simulink model "w2_warplab_trigger_proc"  (Simulink 7.7)
settings: Solver=ode45  StartTime=0.0  StopTime=1000  RelTol=1e-3
InitFcn:
  | w2_warplab_trigger_proc_init
StartFcn:
  | w2_warplab_trigger_proc_init
undefined symbols (not defined in the file or in its folder): gcbh, xlBlockLoadCallback, xlGetNormalizedPeriod
libraries: xbsIndex_r4 x819, simulink x1
(part 1 of 6)
settings Model: Creator=murphpo  LastModifiedBy=mango
settings DebuggingCC: FcnCallInpInsideContextMsg=Enable All

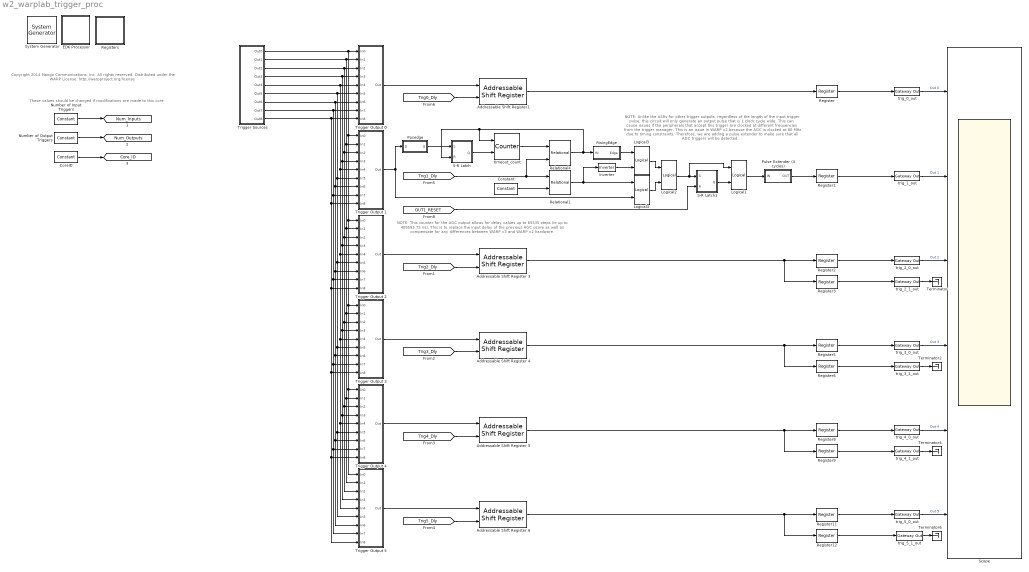
== system w2_warplab_trigger_proc ==
  note: These values should be changed if modifications are made to this core
  note: Copyright 2014 Mango Communications, Inc. All rights reserved.
      |
      | Distributed under the WARP License:
      | http://warpproject.org/license
  note: NOTE:  This counter for the AGC output allows for delay values up to 65535 steps (ie up to 409593.75 ns).
      | This is to replace the input delay of the previous AGC pcore as well as compensate for any differences
      | between WARP v3 and WARP v2 hardware.
  note: NOTE:  Unlike the ASRs for other trigger outputs, regardless of the length of the input trigger pulse, this
      | circuit will only generate an output pulse that is 1 clock cycle wide. This can cause issues if the peripherals
      | that accept this trigger are clocked at different frequencies from the trigger manager.
      |
      | This is an issue in WARP v2 because the AGC is clocked at 80 MHz due to timing constraints.  Therefore,
      | we are adding a pulse extender to make sure that all AGC triggers will be detected.
  " System Generator" : xbsIndex_r4/ System Generator  Tag=genX  SystemSampleTime=-1  xilinxfamily=virtex4  part=xc4vfx100  speed=-11  package=ff1517  synthesis_tool=XST  clock_wrapper=Clock Enables  directory=./trigger_proc  proj_type=Project Navigator  Synth_file=XST Defaults  Impl_file=ISE Defaults  testbench=off  simulink_period=1  sysclk_period=10  dcm_input_clock_period=10  incr_netlist=off  trim_vbits=Everywhere in SubSystem  dbl_ovrd=According to Block Masks  core_generation=According to Block Masks  run_coregen=off  deprecated_control=off  eval_field=0  block_type=sysgen
  Addressable Shift Register {3..6} (4 alike) : xbsIndex_r4/Addressable Shift Register  infer_latency=off  depth=32  initVector=[0]  en=off  dbl_ovrd=off  use_behavioral_HDL=off  Optimization=Resource  block_type=addrsr
      settings: infoedit="Delay of configurable length.  Any element in the delay line can be addressed and driven onto the output port.<br><br>Hardware notes: This block is implemented using SRL16s. If Virtex-4 or Spartan-3 device is used, multiple SRLC16s are cascaded together."
  Addressable Shift Register1 : xbsIndex_r4/Addressable Shift Register  infer_latency=off  depth=32  initVector=[0]  en=off  dbl_ovrd=off  use_behavioral_HDL=off  Optimization=Resource  block_type=addrsr
      settings: infoedit="Delay of configurable length.  Any element in the delay line can be addressed and driven onto the output port.<br><br>Hardware notes: This block is implemented using SRL16s. If Virtex-4 or Spartan-3 device is used, multiple SRLC16s are cascaded together."
  Constant : xbsIndex_r4/Constant  const=0  gui_display_data_type=Fixed-point  arith_type=Unsigned  n_bits=16  bin_pt=0  preci_type=Single  exp_width=8  frac_width=24  explicit_period=off  period=1  equ=P=C  opselect=C  inp2=PCIN>>17  opr=+  inp1=P  carry=CIN  dbl_ovrd=off  block_type=constant
  CoreID : xbsIndex_r4/Constant  const=0  gui_display_data_type=Fixed-point  arith_type=Unsigned  n_bits=8  bin_pt=0  preci_type=Single  exp_width=8  frac_width=24  explicit_period=on  period=1  equ=P=C  opselect=C  inp2=PCIN>>17  opr=+  inp1=P  carry=CIN  dbl_ovrd=off  block_type=constant
  EDK Processor : Subsystem  LoadFcn=xlBlockLoadCallback(gcbh);  mask(Xilinx EDK Processor Block){mode=EDK pcore generation, xmp=, MemVisToProc=<qt bgcolor="#FFFFFF"><div><img src="C:/Xilinx/14.4/ISE_DS/ISE/sysgen/data/images/registerplus.gif"> &lt;&lt;RSSI_PKT_DET_CONFIG&gt;&gt;<br></div><div><img src="C:/Xilinx/14.4/ISE_DS/ISE/sysgen/data/images/registerplus.gif"> &lt;&lt;TRIG_IN_CONF_6&gt;&gt;<br></div><div><img src="C:/Xilinx/14.4/ISE_DS/ISE/sysgen/data/images/registerplus.gif"> &lt;&lt;TRIG_IN_CONF_5&gt;&gt;<br></div><div><img src="C:/Xilinx/14.4/ISE_DS/ISE/sysgen/data/images/registerplus.gif"> &lt;&lt;TRIG_IN_CONF_4&gt;&gt;<br></div><div><img src="C:/Xilinx/14.4/ISE_DS/ISE/sysgen/data/images/registerplus.gif"> &lt;&lt;TRIG_IN_CONF_3&gt;&gt;<br></div><div><img src="C:/Xilinx/14.4/ISE_DS/ISE/sysgen/data/images/registerplus.gif"> &lt;&lt;TRIG_IN_CONF_2&gt;&gt;<br></div><div><img src="C:/Xilinx/14.4/ISE_DS/ISE/sysgen/data/images/registerplus.gif"> &lt;&lt;TRIG_IN_CONF_0&gt;&gt;<br></div><div><img src="C:/Xilinx/14.4/ISE_DS/ISE/sysgen/data/images/registerplus.gif"> &lt;&lt;TRIG_IN_CONF_8&gt;&gt;<br></div><div><img src="C:/Xilinx/14.4/ISE_DS/ISE/sysgen/data/images/registerplus.gif"> &lt;&lt;TRIG_IN_CONF_7&gt;&gt;<br></div><div><img src="C:/Xilinx/14.4/ISE_DS/ISE/sysgen/data/images/registerplus.gif"> &lt;&lt;TRIG_OUT_5_CONF_0&gt;&gt;<br></div><div><img src="C:/Xilinx/14.4/ISE_DS/ISE/sysgen/data/images/registerplus.gif"> &lt;&lt;TRIG_OUT_5_CONF_1&gt;&gt;<br></div><div><img src="C:/Xilinx/14.4/ISE_DS/ISE/sysgen/data/images/registerplus.gif"> &lt;&lt;TRIG_OUT_4_CONF_0&gt;&gt;<br></div><div><img src="C:/Xilinx/14.4/ISE_DS/ISE/sysgen/data/images/registerplus.gif"> &lt;&lt;TRIG_OUT_0_CONF_0&gt;&gt;<br></div><div><img src="C:/Xilinx/14.4/ISE_DS/ISE/sysgen/data/images/registerplus.gif"> &lt;&lt;TRIG_OUT_4_CONF_1&gt;&gt;<br></div><div><img src="C:/Xilinx/14.4/ISE_DS/ISE/sysgen/data/images/registerplus.gif"> &lt;&lt;TRIG_OUT_3_CONF_0&gt;&gt;<br></div><div><img src="C:/Xilinx/14.4/ISE_DS/ISE/sysgen/data/images/registerplus.gif"> &lt;&lt;TRIG_OUT_3_CONF_1&gt;&gt;<br></div><div><img src="C:/Xilinx/14.4/ISE_DS/ISE/sysgen/data/images/registerplus.gif"> &lt;&lt;TRIG_OUT_2_CONF_0&gt;&gt;<br></div><div><img src="C:/Xilinx/14.4/ISE_DS/ISE/sysgen/data/images/registerplus.gif"> &lt;&lt;TRIG_OUT_2_CONF_1&gt;&gt;<br></div><div><img src="C:/Xilinx/14.4/ISE_DS/ISE/sysgen/data/images/registerplus.gif"> &lt;&lt;TRIG_OUT_1_CONF_0&gt;&gt;<br></div><div><img src="C:/Xilinx/14.4/ISE_DS/ISE/sysgen/data/images/registerplus.gif"> &lt;&lt;TRIG_OUT_1_CONF_1&gt;&gt;<br></div><div><img src="C:/Xilinx/14.4/ISE_DS/ISE/sysgen/data/images/registerplus.gif"> &lt;&lt;TRIG_OUT_0_CONF_1&gt;&gt;<br></div><div><img src="C:/Xilinx/14.4/ISE_DS/ISE/sysgen/data/images/registerplus.gif"> &lt;&lt;RSSI_PKT_DET_DURATIONS&gt;&gt;<br></div><div><img src="C:/Xilinx/14.4/ISE_DS/ISE/sysgen/data/images/registerplus.gif"> &lt;&lt;RSSI_PKT_DET_THRESHOLDS&gt;&gt;<br></div><div><img src="C:/Xilinx/14.4/ISE_DS/ISE/sysgen/data/images/registerplus.gif"> &lt;&lt;TRIG_IN_CONF_1&gt;&gt;<br></div><div><img src="C:/Xilinx/14.4/ISE_DS/ISE/sysgen/data/images/registerplus.gif"> &lt;&lt;CORE_INFO&gt;&gt;<br></div><div><img src="C:/Xilinx/14.4/ISE_DS/ISE/sysgen/data/images/registerplus.gif"> &lt;&lt;TRIG_OUT&gt;&gt;<br></div></qt>, AvailableMemories=<empty>, portInterfaceTable={'exposed'=>[],'portdir'=>[],'portname'=>[],'shortname'=>[]}, bus_type_sgadvanced=, bus_type=PLB, baseaddr=0x80000000, baseaddr_lock_sgadvanced=, baseaddr_lock=off, dual_clock_sgadvanced=, dual_clock=on, reg_readback_sgadvanced=, reg_readback=on, ucf_file=, inheritDeviceType_sgadvanced=, inheritDeviceType=off, elf_file=, codebug_sgadvanced=, codebug=on, clock_name=plb, internalPortList={}, resetPolarity=0, memxtable={'mladdr'=>[0.00000000000000000,1.00000000000000000,2.00000000000000000,3.00000000000000000,4.00000000000000000,5.00000000000000000,6.00000000000000000,7.00000000000000000,8.00000000000000000,9.00000000000000000,10.00000000000000000,11.00000000000000000,12.00000000000000000,13.00000000000000000,14.00000000000000000,15.00000000000000000,16.00000000000000000,17.00000000000000000,18.00000000000000000,19.00000000000000000,20.00000000000000000,21.00000000000000000,22.00000000000000000,23.00000000000000000,0.00000000000000000,1.00000000000000000],'mlist'=>['w2_warplab_trigger_proc/Registers/From Register9','w2_warplab_trigger_proc/Registers/From Register8','w2_warplab_trigger_proc/Registers/From Register7','w2_warplab_trigger_proc/Registers/From Register6','w2_warplab_trigger_proc/Registers/From Register5','w2_warplab_trigger_proc/Registers/From Register4','w2_warplab_trigger_proc/Registers/From Register3','w2_warplab_trigger_proc/Registers/From Register24','w2_warplab_trigger_proc/Registers/From Register23','w2_warplab_trigger_proc/Registers/From Register22','w2_warplab_trigger_proc/Registers/From Register21','w2_warplab_trigger_proc/Registers/From Register20','w2_warplab_trigger_proc/Registers/From Register2','w2_warplab_trigger_proc/Registers/From Register19','w2_warplab_trigger_proc/Registers/From Register18','w2_warplab_trigger_proc/Registers/From Register17','w2_warplab_trigger_proc/Registers/From Register16','w2_warplab_trigger_proc/Registers/From Register15','w2_warplab_trigger_proc/Registers/From Register14','w2_warplab_trigger_proc/Registers/From Register13','w2_warplab_trigger_proc/Registers/From Register12','w2_warplab_trigger_proc/Registers/From Register11','w2_warplab_trigger_proc/Registers/From Register10','w2_warplab_trigger_proc/Registers/From Register1','w2_warplab_trigger_proc/Registers/To Register1','w2_warplab_trigger_proc/Registers/To Register'],'mlname'=>['\\'RSSI_PKT_DET_CONFIG\\'','\\'TRIG_IN_CONF_6\\'','\\'TRIG_IN_CONF_5\\'','\\'TRIG_IN_CONF_4\\'','\\'TRIG_IN_CONF_3\\'','\\'TRIG_IN_CONF_2\\'','\\'TRIG_IN_CONF_0\\'','\\'TRIG_IN_CONF_8\\'','\\'TRIG_IN_CONF_7\\'','\\'TRIG_OUT_5_CONF_0\\'','\\'TRIG_OUT_5_CONF_1\\'','\\'TRIG_OUT_4_CONF_0\\'','\\'TRIG_OUT_0_CONF_0\\'','\\'TRIG_OUT_4_CONF_1\\'','\\'TRIG_OUT_3_CONF_0\\'','\\'TRIG_OUT_3_CONF_1\\'','\\'TRIG_OUT_2_CONF_0\\'','\\'TRIG_OUT_2_CONF_1\\'','\\'TRIG_OUT_1_CONF_0\\'','\\'TRIG_OUT_1_CONF_1\\'','\\'TRIG_OUT_0_CONF_1\\'','\\'RSSI_PKT_DET_DURATIONS\\'','\\'RSSI_PKT_DET_THRESHOLDS\\'','\\'TRIG_IN_CONF_1\\'','\\'CORE_INFO\\'','\\'TRIG_OUT\\''],'mlstate'=>[0.00000000000000000,0.00000000000000000,0.00000000000000000,0.00000000000000000,0.00000000000000000,0.00000000000000000,0.00000000000000000,0.00000000000000000,0.00000000000000000,0.00000000000000000,0.00000000000000000,0.00000000000000000,0.00000000000000000,0.00000000000000000,0.00000000000000000,0.00000000000000000,0.00000000000000000,0.00000000000000000,0.00000000000000000,0.00000000000000000,0.00000000000000000,0.00000000000000000,0.00000000000000000,0.00000000000000000,0.00000000000000000,0.00000000000000000]}, procinfo={}, memmapdirty=off, blockname=, xpsintstyle=default, has_advanced_control=0, sggui_pos=-1,-1,-1,-1, block_type=edkprocessor, block_version=2.7, sg_icon_stat=62,64,-1,-1,white,blue,0,07734,right,,[ ],[ ], sg_mask_display=|, sg_list_contents={'table'=>{'AvailableMemories'=>'popup(<empty>)'}}, sg_blockgui_xml=}
      mask sg_mask_display=|
      | fprintf('','COMMENT: begin icon graphics');
      | patch([0 62 62 0 0 ],[0 0 64 64 0 ],[0.77 0.82 0.91 ]);
      | plot([0 62 62 0 0 ],[0 0 64 64 0 ]);
      | patch([13.2 24.76 32.76 40.76 48.76 32.76 21.2 13.2 ],[40.88 40.88 48.88 40.88 48.88 48.88 48.88 40.88 ],[1 1 1 ]);
      | patch([21.2 32.76 24.76 13.2 21.2 ],[32.88 32.88 40.88 40.88 32.88 ],[0.931 0.946 0.973 ]);
      | patch([13.2 24.76 32.76 21.2 13.2 ],[24.88 24.88 32.88 32.88 24.88 ],[1 1 1 ]);
      | patch([21.2 48.76 40.76 32.76 24.76 13.2 21.2 ],[16.88 16.88 24.88 16.88 24.88 24.88 16.88 ],[0.931 0.946 0.973 ]);
      | fprintf('','COMMENT: end icon graphics');
      | fprintf('','COMMENT: begin icon text');
      | fprintf('','COMMENT: end icon text');
      mask prompts: mode "Configure Processor for"; xmp "XPS Project"; MemVisToProc ""; AvailableMemories "Available Memories"; portInterfaceTable ""; bus_type_sgadvanced ""; bus_type "Bus Type"; baseaddr "Base Address"; baseaddr_lock_sgadvanced ""; baseaddr_lock "Lock"; dual_clock_sgadvanced ""; dual_clock "Dual Clocks"; reg_readback_sgadvanced ""; reg_readback "Register Read-Back"; ucf_file "Constraint File"; inheritDeviceType_sgadvanced ""; inheritDeviceType "Inherit Device Type"; elf_file "Initial Program"; codebug_sgadvanced ""; codebug "Enable Co-Debug with Xilinx SDK (Beta)"; clock_name ""; internalPortList ""; resetPolarity ""; memxtable ""; procinfo ""; memmapdirty ""; blockname ""; xpsintstyle ""; has_advanced_control ""; sggui_pos ""; block_type ""; block_version ""; sg_icon_stat ""; sg_mask_display ""; sg_list_contents ""; sg_blockgui_xml ""
      mask help: Xilinx EDK Processor
      mask init:
      | try
      |   tmp_gcb = gcb;
      |   tmp_gcbh = gcbh;
      |   if (strcmp('SysGenIndex',get_param(bdroot(tmp_gcbh),'tag')) && ~isempty(regexp(bdroot(tmp_gcb), '^xbs', 'once')))
      |     return;
      |   end;
      |   xlMungeMaskParams;
      | 
      |   block_type='edkprocessor';
      | 
      |   serialized_declarations = '{''block_type''=>''String''}';
      |   xledkprocessor_init();
      |   ptable_ = xlblockprep(get_param(tmp_gcb, 'MaskWSVariables'));
      |   try
      |     xlBlockMoveCallback(tmp_gcbh);
      |   catch 
      |      clear global xl_updateicon_recursion_guard;
      |   end;
      | catch
      |   global dbgsysgen;
      |   if(~isempty(dbgsysgen) && dbgsysgen)
      |     e = regexprep(lasterr, '\n', '\nError: ');
      |     disp(['Error: While running MaskInit code on block ' tmp_gcb ': ' e]);
      |     error(e);
      |   end
      | end
      settings: CopyFcn=xlProcBlockCopyCallback(gcbh);xlBlockMoveCallback(gcbh);  DeleteFcn=xlDestroyGui(gcbh);  ModelCloseFcn=xlDestroyGui(gcbh);  PreSaveFcn=xlBlockPreSaveCallback(gcbh);  PostSaveFcn=xlBlockPostSaveCallback(gcbh);  DestroyFcn=xlDestroyGui(gcbh);  OpenFcn=bh=gcbh;xlProcBlockCallbacks('populatesharedmemorylistbox',bh);xlOpenGui(bh, 'edkprocessor_gui.xml', @xlProcBlockEnablement, @xlProcBlockAction);  CloseFcn=xlDestroyGui(gcbh);  MoveFcn=xlBlockMoveCallback(gcbh);
      mask Help: eval('');xlDoc('-book','sysgen','-topic','EDK_Processor');
      mask StyleString: popup(EDK pcore generation|HDL netlisting),edit,edit,edit,edit,edit,popup(AXI|PLB),edit,edit,checkbox,edit,checkbox,edit,checkbox,edit,edit,checkbox,edit,edit,checkbox,edit,edit,edit,edit,edit,edit,edit,edit,edit,edit,edit,edit,edit,edit,edit,edit
      mask Display:
      | fprintf('','COMMENT: begin icon graphics');
      | patch([0 62 62 0 0 ],[0 0 64 64 0 ],[0.77 0.82 0.91 ]);
      | plot([0 62 62 0 0 ],[0 0 64 64 0 ]);
      | patch([13.2 24.76 32.76 40.76 48.76 32.76 21.2 13.2 ],[40.88 40.88 48.88 40.88 48.88 48.88 48.88 40.88 ],[1 1 1 ]);
      | patch([21.2 32.76 24.76 13.2 21.2 ],[32.88 32.88 40.88 40.88 32.88 ],[0.931 0.946 0.973 ]);
      | patch([13.2 24.76 32.76 21.2 13.2 ],[24.88 24.88 32.88 32.88 24.88 ],[1 1 1 ]);
      | patch([21.2 48.76 40.76 32.76 24.76 13.2 21.2 ],[16.88 16.88 24.88 16.88 24.88 24.88 16.88 ],[0.931 0.946 0.973 ]);
      | fprintf('','COMMENT: end icon graphics');
      | fprintf('','COMMENT: begin icon text');
      | disp('');
      | 
      | fprintf('','COMMENT: end icon text');
  Inverter : xbsIndex_r4/Inverter  en=off  latency=0  dbl_ovrd=off  block_type=inv
  Logical1 : xbsIndex_r4/Logical  logical_function=OR  inputs=2  en=off  latency=0  precision=Full  arith_type=Unsigned  n_bits=16  bin_pt=0  align_bp=on  dbl_ovrd=off  block_type=logical
  Logical2 : xbsIndex_r4/Logical  logical_function=OR  inputs=2  en=off  latency=0  precision=Full  arith_type=Unsigned  n_bits=16  bin_pt=0  align_bp=on  dbl_ovrd=off  block_type=logical
  Logical3 : xbsIndex_r4/Logical  logical_function=AND  inputs=2  en=off  latency=0  precision=Full  arith_type=Unsigned  n_bits=16  bin_pt=0  align_bp=on  dbl_ovrd=off  block_type=logical
  Logical4 : xbsIndex_r4/Logical  logical_function=AND  inputs=2  en=off  latency=0  precision=Full  arith_type=Unsigned  n_bits=16  bin_pt=0  align_bp=on  dbl_ovrd=off  block_type=logical
  Number of Input Triggers : xbsIndex_r4/Constant  const=9  gui_display_data_type=Fixed-point  arith_type=Unsigned  n_bits=8  bin_pt=0  preci_type=Single  exp_width=8  frac_width=24  explicit_period=on  period=1  equ=P=C  opselect=C  inp2=PCIN>>17  opr=+  inp1=P  carry=CIN  dbl_ovrd=off  block_type=constant
  Number of Output Triggers : xbsIndex_r4/Constant  const=6  gui_display_data_type=Fixed-point  arith_type=Unsigned  n_bits=8  bin_pt=0  preci_type=Single  exp_width=8  frac_width=24  explicit_period=on  period=1  equ=P=C  opselect=C  inp2=PCIN>>17  opr=+  inp1=P  carry=CIN  dbl_ovrd=off  block_type=constant
  Posedge : Subsystem
  Pulse Extender (4 cycles) : Subsystem
  Register{,1..3,5..6,8..9,11..12} (10 alike) : xbsIndex_r4/Register  init=0  rst=off  en=off  dbl_ovrd=off  block_type=register
  Registers : Subsystem
  Relational1 : xbsIndex_r4/Relational  mode=a=b  en=off  latency=0  dbl_ovrd=off  block_type=relational
      settings: xl_area=[5 0 0 9 0 0 0]  block_version=VER_STRING_GOES_HERE
  Relational4 : xbsIndex_r4/Relational  mode=a=b  en=off  latency=0  dbl_ovrd=off  block_type=relational
      settings: xl_area=[5 0 0 9 0 0 0]  block_version=VER_STRING_GOES_HERE
  RisingEdge : Subsystem
  S-R Latch : Subsystem
  S-R Latch1 : Subsystem
  Scope : Scope  NumInputPorts=6
      settings: YMin=-5~-5~-5~-5~-5~-5  YMax=5~5~5~5~5~5
  Terminator{,2,4,6} (4 alike) : Terminator
  Trigger Output 0 : Subsystem
  Trigger Output 1 : Subsystem
  Trigger Output 2 : Subsystem
  Trigger Output 3 : Subsystem
  Trigger Output 4 : Subsystem
  Trigger Output 5 : Subsystem
  Trigger Sources : Subsystem
  timeout_count : xbsIndex_r4/Counter  cnt_type=Free Running  cnt_to=Inf  operation=Up  start_count=0  cnt_by_val=1  arith_type=Unsigned  n_bits=16  bin_pt=0  load_pin=off  rst=on  en=on  explicit_period=on  period=1  dbl_ovrd=off  use_behavioral_HDL=off  implementation=Fabric  use_rpm=off  block_type=counter
      settings: xl_area=[10 18 0 18 0 0 0]  block_version=VER_STRING_GOES_HERE
  trig_0_out : xbsIndex_r4/Gateway Out  inherit_from_input=off  hdl_port=on  timing_constraint=None  locs_specified=off  LOCs={}  UseAsDAC=off  DACChannel='1'  block_type=gatewayout
  trig_1_out : xbsIndex_r4/Gateway Out  inherit_from_input=off  hdl_port=on  timing_constraint=None  locs_specified=off  LOCs={}  UseAsDAC=off  DACChannel='1'  block_type=gatewayout
  trig_2_0_out : xbsIndex_r4/Gateway Out  inherit_from_input=off  hdl_port=on  timing_constraint=None  locs_specified=off  LOCs={}  UseAsDAC=off  DACChannel='1'  block_type=gatewayout
  trig_2_1_out : xbsIndex_r4/Gateway Out  inherit_from_input=off  hdl_port=on  timing_constraint=None  locs_specified=off  LOCs={}  UseAsDAC=off  DACChannel='1'  block_type=gatewayout
  trig_3_0_out : xbsIndex_r4/Gateway Out  inherit_from_input=off  hdl_port=on  timing_constraint=None  locs_specified=off  LOCs={}  UseAsDAC=off  DACChannel='1'  block_type=gatewayout
  trig_3_1_out : xbsIndex_r4/Gateway Out  inherit_from_input=off  hdl_port=on  timing_constraint=None  locs_specified=off  LOCs={}  UseAsDAC=off  DACChannel='1'  block_type=gatewayout
  trig_4_0_out : xbsIndex_r4/Gateway Out  inherit_from_input=off  hdl_port=on  timing_constraint=None  locs_specified=off  LOCs={}  UseAsDAC=off  DACChannel='1'  block_type=gatewayout
  trig_4_1_out : xbsIndex_r4/Gateway Out  inherit_from_input=off  hdl_port=on  timing_constraint=None  locs_specified=off  LOCs={}  UseAsDAC=off  DACChannel='1'  block_type=gatewayout
  trig_5_0_out : xbsIndex_r4/Gateway Out  inherit_from_input=off  hdl_port=on  timing_constraint=None  locs_specified=off  LOCs={}  UseAsDAC=off  DACChannel='1'  block_type=gatewayout
  trig_5_1_out : xbsIndex_r4/Gateway Out  inherit_from_input=off  hdl_port=on  timing_constraint=None  locs_specified=off  LOCs={}  UseAsDAC=off  DACChannel='1'  block_type=gatewayout
  tag scope: Core_ID=global, Num_Inputs=global, Num_Outputs=global
  wires:
  Trigger Sources/1(Out0) -> Trigger Output 0/1(In0), Trigger Output 4/1(In0), Trigger Output 5/1(In0), Trigger Output 3/1(In0), Trigger Output 2/1(In0), Trigger Output 1/1(In0)
  Trigger Sources/2(Out1) -> Trigger Output 0/2(In1), Trigger Output 4/2(In1), Trigger Output 5/2(In1), Trigger Output 3/2(In1), Trigger Output 2/2(In1), Trigger Output 1/2(In1)
  Trigger Sources/3(Out2) -> Trigger Output 0/3(In2), Trigger Output 4/3(In2), Trigger Output 5/3(In2), Trigger Output 3/3(In2), Trigger Output 2/3(In2), Trigger Output 1/3(In2)
  Trigger Sources/4(Out3) -> Trigger Output 0/4(In3), Trigger Output 4/4(In3), Trigger Output 5/4(In3), Trigger Output 3/4(In3), Trigger Output 2/4(In3), Trigger Output 1/4(In3)
  Trigger Sources/5(Out4) -> Trigger Output 0/5(In4), Trigger Output 4/5(In4), Trigger Output 5/5(In4), Trigger Output 3/5(In4), Trigger Output 2/5(In4), Trigger Output 1/5(In4)
  Trigger Sources/6(Out5) -> Trigger Output 0/6(In5), Trigger Output 4/6(In5), Trigger Output 5/6(In5), Trigger Output 3/6(In5), Trigger Output 2/6(In5), Trigger Output 1/6(In5)
  Trigger Sources/7(Out6) -> Trigger Output 0/7(In6), Trigger Output 4/7(In6), Trigger Output 5/7(In6), Trigger Output 3/7(In6), Trigger Output 2/7(In6), Trigger Output 1/7(In6)
  Trigger Sources/8(Out7) -> Trigger Output 0/8(In7), Trigger Output 4/8(In7), Trigger Output 5/8(In7), Trigger Output 3/8(In7), Trigger Output 2/8(In7), Trigger Output 1/8(In7)
  Trigger Output 2/1(Out) -> Addressable Shift Register 3/1
  Addressable Shift Register 3/1 -> Register2/1, Register3/1
  Trigger Output 3/1(Out) -> Addressable Shift Register 4/1
  Addressable Shift Register 4/1 -> Register5/1, Register6/1
  Trigger Output 4/1(Out) -> Addressable Shift Register 5/1
  Addressable Shift Register 5/1 -> Register8/1, Register9/1
  Number of Input Triggers/1 -> [Num_Inputs]
  Number of Output Triggers/1 -> [Num_Outputs]
  CoreID/1 -> [Core_ID]
  Trigger Output 5/1(Out) -> Addressable Shift Register 6/1
  Addressable Shift Register 6/1 -> Register11/1, Register12/1
  trig_0_out/1 -> Scope/1  "Out 0"
  trig_1_out/1 -> Scope/2  "Out 1"
  trig_2_0_out/1 -> Scope/3  "Out 2"
  trig_3_0_out/1 -> Scope/4  "Out 3"
  trig_4_0_out/1 -> Scope/5  "Out 4"
  trig_5_0_out/1 -> Scope/6  "Out 5"
  Trigger Sources/9(Out8) -> Trigger Output 0/9(In8), Trigger Output 4/9(In8), Trigger Output 5/9(In8), Trigger Output 3/9(In8), Trigger Output 2/9(In8), Trigger Output 1/9(In8)
  [Trig0_Dly] -> Addressable Shift Register1/2
  [Trig2_Dly] -> Addressable Shift Register 3/2
  [Trig3_Dly] -> Addressable Shift Register 4/2
  [Trig4_Dly] -> Addressable Shift Register 5/2
  [Trig5_Dly] -> Addressable Shift Register 6/2
  Trigger Output 0/1(Out) -> Addressable Shift Register1/1
  Addressable Shift Register1/1 -> Register/1
  S-R Latch/1(Q) -> timeout_count/2
  timeout_count/1 -> Relational4/1
  Relational4/1 -> timeout_count/1, S-R Latch/2(R), RisingEdge/1(IN)
  [Trig1_Dly] -> Relational4/2, Relational1/1
  Posedge/1(Q) -> S-R Latch/1(S)
  S-R Latch1/1(Q) -> Logical1/2
  Logical1/1 -> Pulse Extender (4 cycles)/1(IN)
  Constant/1 -> Relational1/2
  Relational1/1 -> Logical4/1, Inverter/1
  RisingEdge/1(Edge) -> Logical3/1
  Inverter/1 -> Logical3/2
  Logical3/1 -> Logical2/1
  Logical4/1 -> Logical2/2
  Logical2/1 -> S-R Latch1/1(S), Logical1/1
  Trigger Output 1/1(Out) -> Posedge/1(D), Logical4/2
  [OUT1_RESET] -> S-R Latch1/2(R)
  Register/1 -> trig_0_out/1
  Register1/1 -> trig_1_out/1
  Register2/1 -> trig_2_0_out/1
  Register5/1 -> trig_3_0_out/1
  Register8/1 -> trig_4_0_out/1
  Register11/1 -> trig_5_0_out/1
  Register3/1 -> trig_2_1_out/1
  Register6/1 -> trig_3_1_out/1
  Register9/1 -> trig_4_1_out/1
  Register12/1 -> trig_5_1_out/1
  trig_2_1_out/1 -> Terminator/1
  trig_3_1_out/1 -> Terminator2/1
  trig_4_1_out/1 -> Terminator4/1
  trig_5_1_out/1 -> Terminator6/1
  Pulse Extender (4 cycles)/1(OUT) -> Register1/1
